simulink model "cl_fonp02_syn"  (Simulink 8.1)
settings: Solver=ode3  StartTime=0.0  StopTime=Tend  FixedStep=T  RelTol=1e-3
values from neighbouring files (symbols this model uses):
  Gamma = [-4.33815; 0; 0]    [ss_engine_model.m]
  H = [0 0 -1]    [ss_engine_model.m]
  K1 = myacker(Phi, Gamma, z1)    [cl_fonp02.m]    (also in cl_fonp03.m = place(Phi, Gamma, z1))
  n = length(Phi)    [cl_fonp02.m]    (also in cl_fonp03.m; direct_design.m = order; sylvester.m = max(nA, nB) - 1)
  Phi = [0 0 -0.00237 ... (first row only)    [ss_engine_model.m]
  T = 1    [cd_plot1.m]    (also in cd_plot2.m; cl_ff01.m; cl_fonp02.m; cl_fonp03.m)
  x0 = [1; zeros(length(sysX.a) - 1, 1)]    [cl_ff01.m]    (also in cl_fonp02.m = rpm_lo*H; cl_fonp03.m = rpm_lo*H; lsim1.m = false)
libraries: simulink x1
settings Model: Creator=jmahler  LastModifiedBy=jmahler
settings DataIOCC: SignalLoggingSaveFormat=Dataset
settings OptimizationCC: ExpressionDepthLimit=128
settings DebuggingCC: FcnCallInpInsideContextMsg=EnableAllAsError
settings GRTTargetCC: CombineOutputUpdateFcns=on  GRTInterface=off

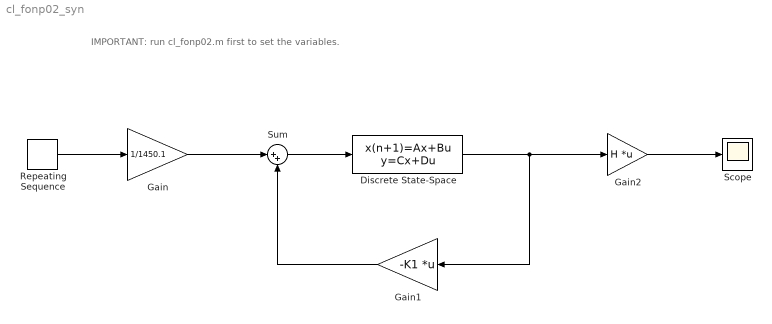
== system cl_fonp02_syn ==
  note: IMPORTANT: run cl_fonp02.m first to set the variables.
  Discrete State-Space : DiscreteStateSpace  A=Phi  B=Gamma  C=eye(n)  D=zeros(n,1)  X0=x0  SampleTime=T
  Gain : Gain  Gain=1/1450.1
  Gain1 : Gain  Gain=-K1  Multiplication=Matrix(K*u)
  Gain2 : Gain  Gain=H  Multiplication=Matrix(K*u)  SampleTime=T
  Repeating Sequence : simulink/Sources/Repeating Sequence  rep_seq_t=t1  rep_seq_y=u
  Scope : Scope
  Sum : Sum  Inputs=|++
  wires:
  Sum/1 -> Discrete State-Space/1
  Gain/1 -> Sum/1
  Gain1/1 -> Sum/2
  Gain2/1 -> Scope/1
  Discrete State-Space/1 -> Gain2/1, Gain1/1
  Repeating Sequence/1 -> Gain/1
